simulink model "w2_cc"  (R2020b)
settings: Solver=ode45  StartTime=0.0  StopTime=10  RelTol=1e-3
model workspace (MAT data in the model file):
  Ki = 40
  Kp = 1000
  b = 50
  m = 1000
  u = 500
settings Model: DataDictionary=W2_cc.sldd  Creator=mluser  LastModifiedBy=mluser

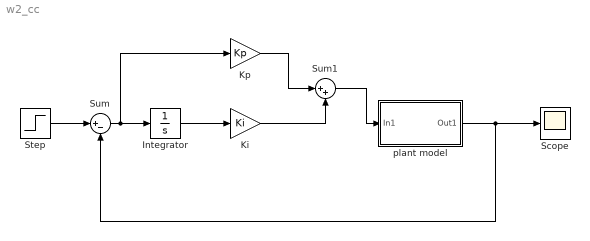
== system w2_cc ==
  Integrator : Integrator
  Ki : Gain  Gain=Ki
  Kp : Gain  Gain=Kp
  Scope : Scope
  Step : Step  Time=0  After=u  SampleTime=0
  Sum : Sum  Inputs=|+-
  Sum1 : Sum  Inputs=|++
  plant model : Subsystem
  wires:
  Sum/1 -> Kp/1, Integrator/1
  plant model/1(Out1) -> Scope/1, Sum/2
  Sum1/1 -> plant model/1(In1)
  Ki/1 -> Sum1/2
  Integrator/1 -> Ki/1
  Kp/1 -> Sum1/1
  Step/1 -> Sum/1

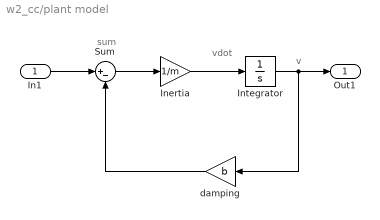
== system w2_cc/plant model ==
  note: vdot
  note: sum
  note: v
  In1 : Inport
  Inertia : Gain  Gain=1/m
  Integrator : Integrator
  Sum : Sum  Inputs=|+-
  damping : Gain  Gain=b
  Out1 : Outport
  wires:
  In1/1 -> Sum/1
  Sum/1 -> Inertia/1
  Inertia/1 -> Integrator/1
  damping/1 -> Sum/2
  Integrator/1 -> Out1/1, damping/1
